simulink model "rest_spike_bistability_original"  (R2015a)
settings: Solver=ode45  StartTime=0.0  StopTime=10000  RelTol=1e-3
values from neighbouring files (symbols this model uses):
  alpha = 0.25    [fast_nullcline_winged_cusp.m]    (also in relay_model_bistability.m; relay_model_bistability2.m)
  beta = 0.5    [fast_nullcline_winged_cusp.m]    (also in relay_model_bistability.m; relay_model_bistability2.m = 0.25)
  delta = 0.5    [fast_nullcline_winged_cusp.m]    (also in relay_model_bistability.m = 0.3; relay_model_bistability2.m = 0.3)
  gamma = 0.5    [fast_nullcline_winged_cusp.m]    (also in relay_model_bistability.m = 1; relay_model_bistability2.m = 1)
  ts = 1    [fast_nullcline_winged_cusp.m]    (also in relay_model_bistability.m = 0.5; relay_model_bistability2.m)
settings Model: CovModelRefEnable=off  Creator=rajiv  LastModifiedBy=ra428
settings DataIOCC: SaveFormat=Dataset
settings HardwareCC: ProdBitPerPointer=64  ProdLargestAtomicFloat=Float  ProdIntDivRoundTo=Zero  ProdEndianess=LittleEndian  ProdHWDeviceType=Specified
settings GRTTargetCC: GeneratePreprocessorConditionals=Use local settings

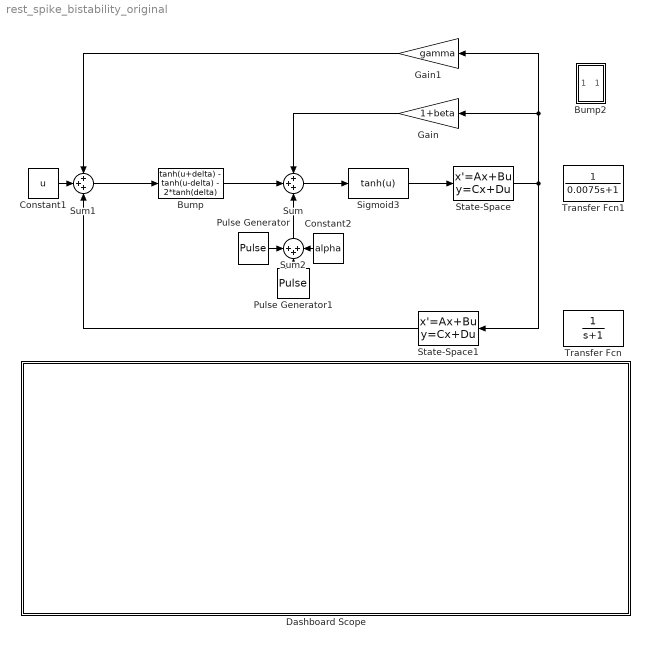
== system rest_spike_bistability_original ==
  Bump : Fcn  Expr="tanh(u+delta) -  tanh(u-delta) - 2*tanh(delta)"
  Bump2 : Subsystem
  Constant1 : Constant  Value=u
  Constant2 : Constant  Value=alpha
  Dashboard Scope : Subsystem  DialogController=hmiCreateDDGDialog  IsWebBlock=on  mask(MWDashboardBlock){webBlockId=290fb283-b992-4812-92b1-e9dbbb5c61cf, webBlockType=sdiscope, ShowInitialText=on, HMISrcModelName=rest_spike_bistability_original}
      mask prompts: webBlockId "WebBlock Id"; webBlockType "WebBlock Type"; HMISrcModelName "Source Model"
      mask Help: helpview([docroot '/mapfiles/simulink.map'], 'hmi_scope')
      mask Display:
      | if strcmp(get_param(bdroot(gcb),'BlockDiagramType'), 'library')
      |     image([(matlabroot) '/toolbox/simulink/hmi/icons/DashboardScope.png']);
      | end
  Gain : Gain  Gain=1+beta
  Gain1 : Gain  Gain=gamma
  Pulse Generator : DiscretePulseGenerator  PulseType=Time based  Period=10000  PhaseDelay=4000
  Pulse Generator1 : DiscretePulseGenerator  PulseType=Time based  Amplitude=-1  Period=10000  PhaseDelay=7000
  Sigmoid3 : Fcn  Expr=tanh(u)
  State-Space : StateSpace  A=-1/tf  B=1/tf  D=0  X0=-1
  State-Space1 : StateSpace  A=-1/ts  B=1/ts  D=0  X0=-1
  Sum : Sum  Inputs=+++
  Sum1 : Sum  Inputs=+++
  Sum2 : Sum  Inputs=+++
  Transfer Fcn : TransferFcn  Denominator=[1 1]
  Transfer Fcn1 : TransferFcn  Denominator=[0.0075 1]
  wires:
  Sum/1 -> Sigmoid3/1
  Gain/1 -> Sum/1
  State-Space1/1 -> Sum1/3
  Gain1/1 -> Sum1/1
  Constant1/1 -> Sum1/2
  Sigmoid3/1 -> State-Space/1
  State-Space/1 -> State-Space1/1, Gain/1, Gain1/1
  Constant2/1 -> Sum2/3
  Pulse Generator/1 -> Sum2/1
  Sum2/1 -> Sum/3
  Pulse Generator1/1 -> Sum2/2
  Bump/1 -> Sum/2
  Sum1/1 -> Bump/1

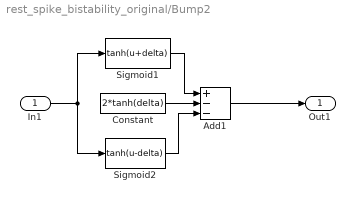
== system rest_spike_bistability_original/Bump2 ==
  In1 : Inport
  Add1 : Sum  Inputs=+--
  Constant : Constant  Value=2*tanh(delta)
  Sigmoid1 : Fcn  Expr=tanh(u+delta)
  Sigmoid2 : Fcn  Expr=tanh(u-delta)
  Out1 : Outport
  wires:
  Sigmoid2/1 -> Add1/3
  Constant/1 -> Add1/2
  Add1/1 -> Out1/1
  Sigmoid1/1 -> Add1/1
  In1/1 -> Sigmoid2/1, Sigmoid1/1

== system rest_spike_bistability_original/Dashboard Scope ==
